simulink model "set_rcs"  (R2020a)
settings: Solver=FixedStepDiscrete  StartTime=0.0  StopTime=10.0  RelTol=1e-3
settings Model: Creator=thomas  LastModifiedBy=thomas

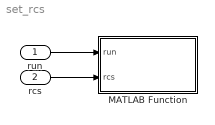
== system set_rcs ==
  run : Inport  OutDataTypeStr=boolean
  rcs : Inport  Port=2  OutDataTypeStr=boolean
  MATLAB Function : MATLAB Function  TreatAsAtomicUnit=on
  wires:
  rcs/1 -> MATLAB Function/2(rcs)
  run/1 -> MATLAB Function/1(run)

== matlab function set_rcs/MATLAB Function ==
  data: run input; rcs input boolean
function set_rcs(run, rcs)
    coder.extrinsic('evalin');
    if run
        evalin('base', sprintf('vessel_control.setRCS(%u);', uint8(rcs)));
    end
end
